simulink library "ilcPathOptThrTen_cl"  (R2020a)
settings: Solver=VariableStepAuto  StartTime=0.0  StopTime=10.0  RelTol=1e-3
undefined symbols (not defined in the file or in its folder): hiLvlCtrl, initializeBussesFromBlock
libraries: stopwatch_ul x2, ilcPhase_cl x1, ilcUpdate_cl x1, runningAvg_ul x1, ilcPathOpt_cl x1
settings Model: Creator=mcobb  LastModifiedBy=adabney
settings DataIOCC: ReturnWorkspaceOutputs=off
settings DebuggingCC: ArithmeticOperatorsInVariantConditions=warning
settings SFSimCC: CustomCodeUndefinedFunction=UseInterfaceOnly

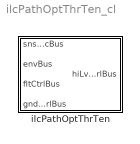
== system ilcPathOptThrTen_cl ==
  ilcPathOptThrTen : Subsystem  LoadFcn=initializeBussesFromBlock(gcb)  InitFcn=initializeBussesFromBlock(gcb)  StartFcn=initializeBussesFromBlock(gcb)  mask{ctrl=hiLvlCtrl}
      mask prompts: ctrl "Controller Object"
      settings: MinAlgLoopOccurrences=on

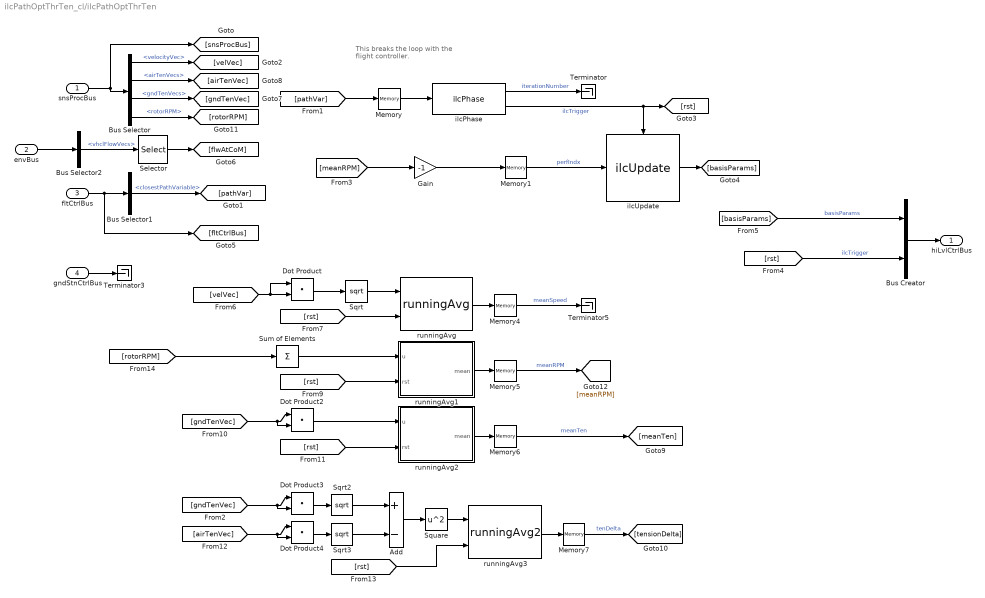
== system ilcPathOptThrTen_cl/ilcPathOptThrTen ==
  note: This breaks the loop
      | with the flight controller.
  snsProcBus : Inport  OutDataTypeStr=Bus: sensorsProcessingBus
  envBus : Inport  Port=2  OutDataTypeStr=Bus: envBus
  fltCtrlBus : Inport  Port=3  OutDataTypeStr=Bus: fltCtrlBus
  gndStnCtrlBus : Inport  Port=4  OutDataTypeStr=Bus: gndStnCtrlBus
  Add : Sum  Inputs=+-
  Bus Creator : BusCreator  Inputs=2  OutDataTypeStr=Bus: hiLvlCtrlBus
  Bus Selector : BusSelector  OutputSignals=velocityVec,airTenVecs,gndTenVecs,rotorRPM
  Bus Selector1 : BusSelector  OutputSignals=closestPathVariable
  Bus Selector2 : BusSelector  OutputSignals=vhclFlowVecs
  Dot Product{,2..4} (4 alike) : DotProduct  InputSameDT=on  OutDataTypeStr=Inherit: Inherit via internal rule
  Gain : Gain  Gain=-1
  Memory{,1,4..7} (6 alike) : Memory
  Selector : Selector  NumberOfDimensions=2  InputPortWidth=3  IndexOptions=Select all,Index vector (dialog)  Indices=[1 3],5  OutputSizes=1,1
  Sqrt : Sqrt  SaturateOnIntegerOverflow=on
  Sqrt2 : Sqrt  SaturateOnIntegerOverflow=on
  Sqrt3 : Sqrt  SaturateOnIntegerOverflow=on
  Square : Math  Operator=square  SaturateOnIntegerOverflow=on
  Sum of Elements : Sum  Inputs=+
  Terminator : Terminator
  Terminator3 : Terminator
  Terminator5 : Terminator
  ilcPhase : ilcPhase_cl/ilcPhase  upperLim=ctrl.pathVarUpperLim.Value  lowerLim=ctrl.pathVarLowerLim.Value  numInitLaps=ctrl.numInitLaps.Value
  ilcUpdate : ilcUpdate_cl/ilcUpdate  initBasisParams=ctrl.initBasisParams.Value  lrn=ctrl.learningGain.Value  AdaptationParameter=ctrl.forgettingFactor.Value  trstRgn=ctrl.trustRegion.Value  amp=ctrl.excitationAmp.Value  enableVec=ctrl.optEnable.Value
  runningAvg : runningAvg_ul/runningAvg  SystemSampleTime=-1  Latency=0  AutoFrameSizeCalculation=off
  runningAvg1 : Subsystem
  runningAvg2 : Subsystem
  runningAvg3 : ilcPathOpt_cl/ilcPathOpt/runningAvg2  SystemSampleTime=-1  Latency=0  AutoFrameSizeCalculation=off
  hiLvlCtrlBus : Outport  OutDataTypeStr=Bus: hiLvlCtrlBus  VectorParamsAs1DForOutWhenUnconnected=off
  wires:
  Memory1/1 -> ilcUpdate/1  "perfIndx"
  snsProcBus/1 -> [snsProcBus], Bus Selector/1
  envBus/1 -> Bus Selector2/1
  fltCtrlBus/1 -> [fltCtrlBus], Bus Selector1/1
  gndStnCtrlBus/1 -> Terminator3/1
  ilcUpdate/1 -> [basisParams]
  Bus Selector1/1 -> [pathVar]  "<closestPathVariable>"
  ilcPhase/2 -> [rst], ilcUpdate/Trigger  "ilcTrigger"
  [meanRPM] -> Gain/1
  ilcPhase/1 -> Terminator/1  "iterationNumber"
  [pathVar] -> Memory/1
  [basisParams] -> Bus Creator/1  "basisParams"
  Bus Selector/1 -> [velVec]  "<velocityVec>"
  [velVec] -> Dot Product/1, Dot Product/2
  [rst] -> runningAvg/2
  runningAvg/1 -> Memory4/1
  Memory4/1 -> Terminator5/1  "meanSpeed"
  Dot Product/1 -> Sqrt/1
  Sqrt/1 -> runningAvg/1
  Bus Selector2/1 -> Selector/1  "<vhclFlowVecs>"
  Selector/1 -> [flwAtCoM]
  Sum of Elements/1 -> runningAvg1/1(u)
  Memory5/1 -> [meanRPM]  "meanRPM"
  runningAvg1/1(mean) -> Memory5/1
  [rst] -> runningAvg1/2(rst)
  Bus Selector/3 -> [gndTenVec]  "<gndTenVecs>"
  [gndTenVec] -> Dot Product2/2, Dot Product2/1
  [rst] -> runningAvg2/2(rst)
  runningAvg2/1(mean) -> Memory6/1
  Memory6/1 -> [meanTen]  "meanTen"
  Dot Product2/1 -> runningAvg2/1(u)
  Bus Creator/1 -> hiLvlCtrlBus/1
  [rst] -> Bus Creator/2  "ilcTrigger"
  Memory/1 -> ilcPhase/1
  Bus Selector/2 -> [airTenVec]  "<airTenVecs>"
  [gndTenVec] -> Dot Product3/2, Dot Product3/1
  Dot Product3/1 -> Sqrt2/1
  Dot Product4/1 -> Sqrt3/1
  [airTenVec] -> Dot Product4/2, Dot Product4/1
  Sqrt2/1 -> Add/1
  Sqrt3/1 -> Add/2
  Add/1 -> Square/1
  runningAvg3/1 -> Memory7/1
  Memory7/1 -> [tensionDelta]  "tenDelta"
  Square/1 -> runningAvg3/1
  [rst] -> runningAvg3/2
  Bus Selector/4 -> [rotorRPM]  "<rotorRPM>"
  [rotorRPM] -> Sum of Elements/1
  Gain/1 -> Memory1/1

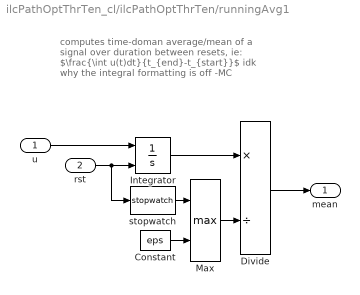
== system ilcPathOptThrTen_cl/ilcPathOptThrTen/runningAvg1 ==
  note: computes time-doman average/mean of a
      | signal over duration between resets, ie:
      | $\frac{\int u(t)dt}{t_{end}-t_{start}}$
      | idk why the integral formatting is off -MC
  u : Inport
  rst : Inport  Port=2
  Constant : Constant  Value=eps
  Divide : Product  Inputs=*/
  Integrator : Integrator  ExternalReset=rising
  Max : MinMax  Function=max  Inputs=2
  stopwatch : stopwatch_ul/stopwatch  SystemSampleTime=-1  Latency=0  AutoFrameSizeCalculation=off
  mean : Outport  VectorParamsAs1DForOutWhenUnconnected=off
  wires:
  Integrator/1 -> Divide/1
  u/1 -> Integrator/1
  stopwatch/1 -> Max/1
  Divide/1 -> mean/1
  Constant/1 -> Max/2
  Max/1 -> Divide/2
  rst/1 -> stopwatch/1, Integrator/2

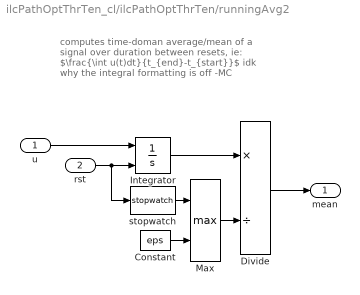
== system ilcPathOptThrTen_cl/ilcPathOptThrTen/runningAvg2 ==
  note: computes time-doman average/mean of a
      | signal over duration between resets, ie:
      | $\frac{\int u(t)dt}{t_{end}-t_{start}}$
      | idk why the integral formatting is off -MC
  u : Inport
  rst : Inport  Port=2
  Constant : Constant  Value=eps
  Divide : Product  Inputs=*/
  Integrator : Integrator  ExternalReset=rising
  Max : MinMax  Function=max  Inputs=2
  stopwatch : stopwatch_ul/stopwatch  SystemSampleTime=-1  Latency=0  AutoFrameSizeCalculation=off
  mean : Outport  VectorParamsAs1DForOutWhenUnconnected=off
  wires:
  rst/1 -> Integrator/2, stopwatch/1
  Max/1 -> Divide/2
  Constant/1 -> Max/2
  Divide/1 -> mean/1
  stopwatch/1 -> Max/1
  u/1 -> Integrator/1
  Integrator/1 -> Divide/1
